simulink model "mmixedts"  (Simulink 7.5)
settings: Solver=FixedStepDiscrete  SolverMode=SingleTasking  StartTime=0.0  StopTime=10.0  RelTol=1e-3
PreLoadFcn:
  | load dmixtsbus
settings Model: Creator=mshakeri  LastModifiedBy=byu  ExtModeAutoUpdateStatusClock=off
settings OptimizationCC: InlineParams=on  InitFltsAndDblsToZero=on
settings DebuggingCC: SaveWithParameterizedLinksMsg=none  SignalResolutionControl=TryResolveAllWithWarning  MultiTaskDSMMsg=warning  MultiTaskCondExecSysMsg=none  UnconnectedInputMsg=none  UnconnectedOutputMsg=none  UnconnectedLineMsg=none  SFUnexpectedBacktrackingDiag=warning  SFNoUnconditionalDefaultTransitionDiag=warning
settings RTWCC: IncludeERTFirstTime=on
settings GRTTargetCC: TargetFcnLib=ansi_tfl_tmw.mat

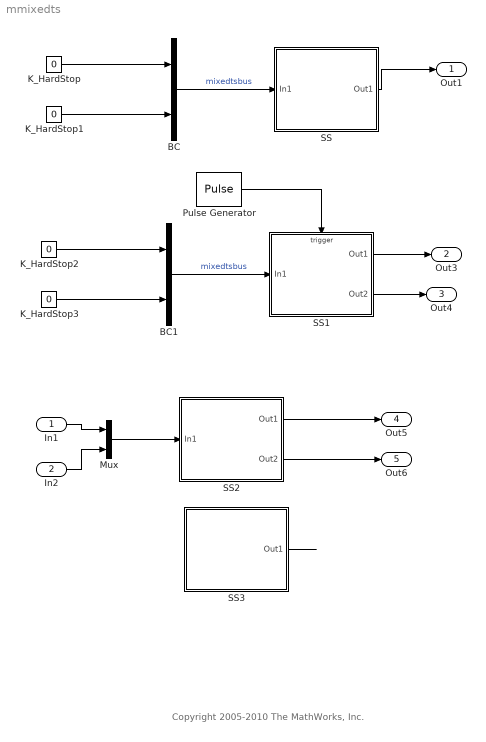
== system mmixedts ==
  note: Copyright 2005-2010 The MathWorks, Inc.
  In1 : Inport  OutDataType=sfix(16)  OutScaling=2^0
  In2 : Inport  Port=2  OutDataType=sfix(16)  OutScaling=2^0
  BC : BusCreator  Inputs=2  UseBusObject=on
      settings: BusObject=mixedtsbus
  BC1 : BusCreator  Inputs=2  UseBusObject=on
      settings: BusObject=sametsbus
  K_HardStop : Constant  Value=0  OutDataTypeMode=boolean  OutDataType=sfix(16)  OutScaling=2^0  OutDataTypeStr=boolean  SampleTime=1
  K_HardStop1 : Constant  Value=0  OutDataTypeMode=boolean  OutDataType=sfix(16)  OutScaling=2^0  OutDataTypeStr=boolean  SampleTime=2
  K_HardStop2 : Constant  Value=0  OutDataTypeMode=boolean  OutDataType=sfix(16)  OutScaling=2^0  OutDataTypeStr=boolean  SampleTime=1
  K_HardStop3 : Constant  Value=0  OutDataTypeMode=boolean  OutDataType=sfix(16)  OutScaling=2^0  OutDataTypeStr=boolean  SampleTime=1
  Mux : Mux  Inputs=2
  Pulse Generator : DiscretePulseGenerator  Amplitude=1  Period=2  PulseWidth=1  PhaseDelay=0  SampleTime=1
  SS : Subsystem  TreatAsAtomicUnit=on
  SS1 : Subsystem  TreatAsAtomicUnit=on
  SS2 : Subsystem  TreatAsAtomicUnit=on
  SS3 : Subsystem  TreatAsAtomicUnit=on
  Out1 : Outport  OutDataType=sfix(16)  OutScaling=2^0
  Out3 : Outport  Port=2  OutDataType=sfix(16)  OutScaling=2^0
  Out4 : Outport  Port=3  OutDataType=sfix(16)  OutScaling=2^0
  Out5 : Outport  Port=4  OutDataType=sfix(16)  OutScaling=2^0
  Out6 : Outport  Port=5  OutDataType=sfix(16)  OutScaling=2^0
  wires:
  K_HardStop/1 -> BC/1
  K_HardStop1/1 -> BC/2
  BC/1 -> SS/1(In1)  "mixedtsbus"
  SS/1(Out1) -> Out1/1
  K_HardStop2/1 -> BC1/1
  K_HardStop3/1 -> BC1/2
  BC1/1 -> SS1/1(In1)  "mixedtsbus"
  SS1/1(Out1) -> Out3/1
  SS1/2(Out2) -> Out4/1
  Pulse Generator/1 -> SS1/Trigger
  In1/1 -> Mux/1
  In2/1 -> Mux/2
  Mux/1 -> SS2/1(In1)
  SS2/1(Out1) -> Out5/1
  SS2/2(Out2) -> Out6/1
  SS3/1(Out1) -> ?

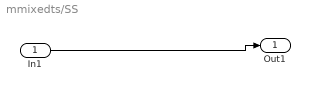
== system mmixedts/SS ==
  In1 : Inport  OutDataType=sfix(16)  OutScaling=2^0
  Out1 : Outport  OutDataType=sfix(16)  OutScaling=2^0
  wires:
  In1/1 -> Out1/1

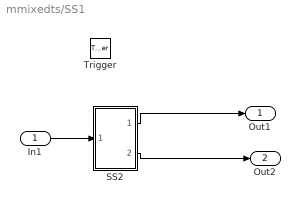
== system mmixedts/SS1 ==
  In1 : Inport  OutDataType=sfix(16)  OutScaling=2^0
  Trigger : TriggerPort
  SS2 : Subsystem  TreatAsAtomicUnit=on
  Out1 : Outport  OutDataType=sfix(16)  OutScaling=2^0
  Out2 : Outport  Port=2  OutDataType=sfix(16)  OutScaling=2^0
  wires:
  SS2/2(Out2) -> Out2/1
  SS2/1(Out1) -> Out1/1
  In1/1 -> SS2/1(In1)

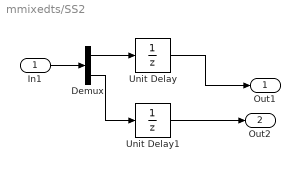
== system mmixedts/SS2 ==
  In1 : Inport  OutDataType=sfix(16)  OutScaling=2^0
  Demux : Demux  Outputs=2
  Unit Delay : UnitDelay
  Unit Delay1 : UnitDelay  SampleTime=2
  Out1 : Outport  OutDataType=sfix(16)  OutScaling=2^0
  Out2 : Outport  Port=2  OutDataType=sfix(16)  OutScaling=2^0
  wires:
  In1/1 -> Demux/1
  Demux/1 -> Unit Delay/1
  Demux/2 -> Unit Delay1/1
  Unit Delay/1 -> Out1/1
  Unit Delay1/1 -> Out2/1

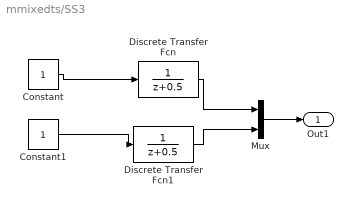
== system mmixedts/SS3 ==
  Constant : Constant  OutDataType=sfix(16)  OutScaling=2^0  SampleTime=1
  Constant1 : Constant  OutDataType=sfix(16)  OutScaling=2^0  SampleTime=2
  Discrete Transfer Fcn : DiscreteTransferFcn
  Discrete Transfer Fcn1 : DiscreteTransferFcn  SampleTime=2
  Mux : Mux  Inputs=2
  Out1 : Outport  OutDataType=sfix(16)  OutScaling=2^0
  wires:
  Constant1/1 -> Discrete Transfer Fcn1/1
  Constant/1 -> Discrete Transfer Fcn/1
  Discrete Transfer Fcn/1 -> Mux/1
  Discrete Transfer Fcn1/1 -> Mux/2
  Mux/1 -> Out1/1

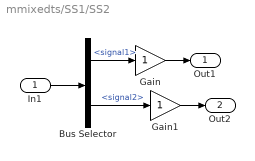
== system mmixedts/SS1/SS2 ==
  In1 : Inport  OutDataType=sfix(16)  OutScaling=2^0
  Bus Selector : BusSelector  OutputSignals=signal1,signal2
  Gain : Gain  ParameterDataType=sfix(16)  ParameterScaling=2^0  OutDataType=sfix(16)  OutScaling=2^0
  Gain1 : Gain  ParameterDataType=sfix(16)  ParameterScaling=2^0  OutDataType=sfix(16)  OutScaling=2^0
  Out1 : Outport  OutDataType=sfix(16)  OutScaling=2^0
  Out2 : Outport  Port=2  OutDataType=sfix(16)  OutScaling=2^0
  wires:
  Bus Selector/2 -> Gain1/1  "<signal2>"
  Bus Selector/1 -> Gain/1  "<signal1>"
  In1/1 -> Bus Selector/1
  Gain/1 -> Out1/1
  Gain1/1 -> Out2/1
